simulink model "Q7_Cascade_Realization"  (R2020b)
settings: Solver=VariableStepAuto  StartTime=0.0  StopTime=10.0  RelTol=1e-3
values from neighbouring files (symbols this model uses):
  a0 = 1.0    [data_dict.sldd]
  a1 = -2.0    [data_dict.sldd]
  a2 = -1.0    [data_dict.sldd]
  a3 = 1.0    [data_dict.sldd]
  a4 = 1.0    [data_dict.sldd]
  a5 = -1.0    [data_dict.sldd]
libraries: simulink x1
settings Model: DataDictionary=data_dict.sldd  Creator=Shree  LastModifiedBy=Shree

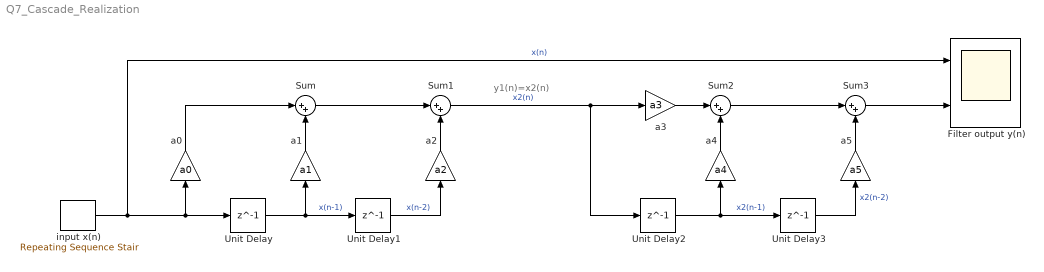
== system Q7_Cascade_Realization ==
  note: y1(n)=x2(n)
  Filter output y(n) : Scope  NumInputPorts=2
  Sum{,1..3} (4 alike) : Sum  Inputs=|++
  Unit Delay{,1..3} (4 alike) : Delay  DelayLength=1  InitialCondition=0
  a0 : Gain  Gain=a0
  a1 : Gain  Gain=a1
  a2 : Gain  Gain=a2
  a3 : Gain  Gain=a3
  a4 : Gain  Gain=a4
  a5 : Gain  Gain=a5
  input x(n) : simulink/Sources/Repeating Sequence Stair  OutValues=[3 1 4 2 1].'  tsamp=-1  OutMin=[]  OutMax=[]  OutDataTypeStr=double  OutputDataTypeScalingMode=double  OutDataType=fixdt(0,8)  ConRadixGroup=Best Precision: Vector-wise  OutScaling=2^-12
  wires:
  input x(n)/1 -> Filter output y(n)/1, Unit Delay/1, a0/1  "x(n)"
  Unit Delay/1 -> a1/1, Unit Delay1/1  "x(n-1)"
  Unit Delay1/1 -> a2/1  "x(n-2)"
  Sum/1 -> Sum1/1
  Sum1/1 -> a3/1, Unit Delay2/1  "x2(n)"
  Unit Delay2/1 -> a4/1, Unit Delay3/1  "x2(n-1)"
  Sum2/1 -> Sum3/1
  Unit Delay3/1 -> a5/1  "x2(n-2)"
  Sum3/1 -> Filter output y(n)/2
  a0/1 -> Sum/1
  a1/1 -> Sum/2
  a2/1 -> Sum1/2
  a4/1 -> Sum2/2
  a5/1 -> Sum3/2
  a3/1 -> Sum2/1
